simulink model "dus4_3"  (R2014a)
settings: Solver=FixedStepDiscrete  StartTime=0.0  StopTime=10.0  FixedStep=0.1  RelTol=1e-3
settings Model: Creator=yoshi12  LastModifiedBy=yoshi12

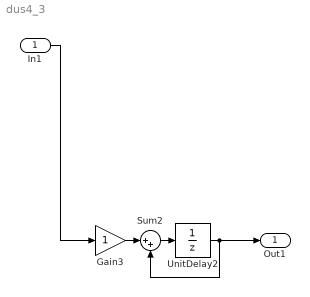
== system dus4_3 ==
  In1 : Inport
  Gain3 : Gain
  Sum2 : Sum  Inputs=|++
  UnitDelay2 : UnitDelay  SampleTime=-1
  Out1 : Outport
  wires:
  In1/1 -> Gain3/1
  Gain3/1 -> Sum2/1
  UnitDelay2/1 -> Out1/1, Sum2/2
  Sum2/1 -> UnitDelay2/1
